simulink model "untitled55"  (R2016a)
settings: Solver=VariableStepAuto  StartTime=0.0  StopTime=1  RelTol=1e-3
settings Model: Creator=liaoyiqi  LastModifiedBy=liaoyiqi

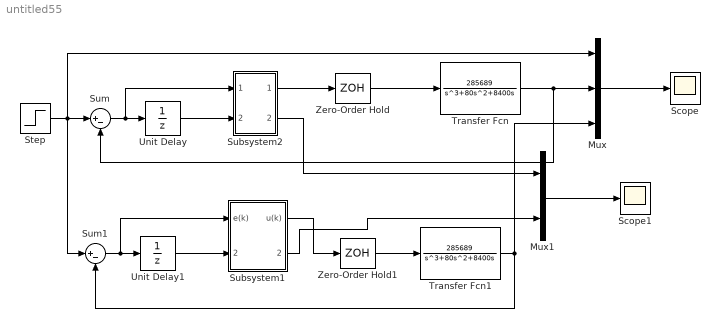
== system untitled55 ==
  Mux : Mux  Inputs=3
  Mux1 : Mux  Inputs=2
  Scope : Scope
  Scope1 : Scope
  Step : Step  Time=0  After=30  SampleTime=0
  Subsystem1 : Subsystem
  Subsystem2 : Subsystem
  Sum : Sum  Inputs=|+-
  Sum1 : Sum  Inputs=|+-
  Transfer Fcn : TransferFcn  Numerator=[285689]  Denominator=[1 80 8400 0]
  Transfer Fcn1 : TransferFcn  Numerator=[285689]  Denominator=[1 80 8400 0]
  Unit Delay : UnitDelay  SampleTime=0.001
  Unit Delay1 : UnitDelay  SampleTime=0.001
  Zero-Order Hold : ZeroOrderHold  SampleTime=0.001
  Zero-Order Hold1 : ZeroOrderHold  SampleTime=0.001
  wires:
  Step/1 -> Mux/1, Sum1/1, Sum/1
  Sum/1 -> Subsystem2/1(In1), Unit Delay/1
  Unit Delay/1 -> Subsystem2/2(In2)
  Zero-Order Hold/1 -> Transfer Fcn/1
  Mux/1 -> Scope/1
  Transfer Fcn/1 -> Sum/2, Mux/2
  Sum1/1 -> Subsystem1/1("e(k) "), Unit Delay1/1
  Subsystem2/1(Out1) -> Zero-Order Hold/1
  Unit Delay1/1 -> Subsystem1/2(e(k-1))
  Zero-Order Hold1/1 -> Transfer Fcn1/1
  Mux1/1 -> Scope1/1
  Subsystem2/2(Out2) -> Mux1/1
  Transfer Fcn1/1 -> Sum1/2, Mux/3
  Subsystem1/1(u(k)) -> Zero-Order Hold1/1
  Subsystem1/2(Out2) -> Mux1/2

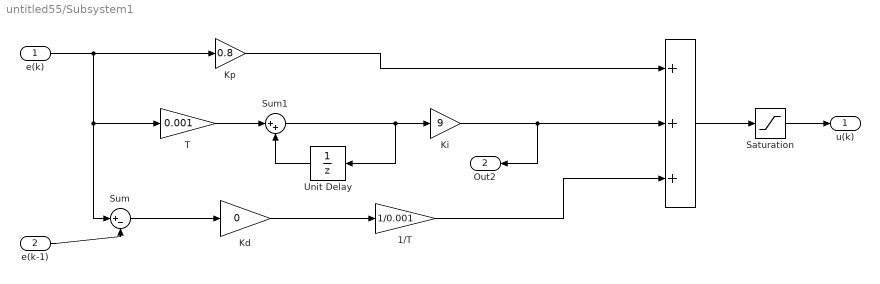
== system untitled55/Subsystem1 ==
  "e(k) " : Inport
  e(k-1) : Inport  Port=2
  " " : Sum  Inputs=+++
  1/T : Gain  Gain=1/0.001
  Kd : Gain  Gain=0
  Ki : Gain  Gain=9
  Kp : Gain  Gain=0.8
  Saturation : Saturate  UpperLimit=10  LowerLimit=-10
  Sum : Sum  Inputs=|+-
  Sum1 : Sum  Inputs=|++
  T : Gain  Gain=0.001
  Unit Delay : UnitDelay  SampleTime=0.001
  u(k) : Outport
  Out2 : Outport  Port=2
  wires:
  Sum1/1 -> Unit Delay/1, Ki/1
  Kd/1 -> 1/T/1
  Sum/1 -> Kd/1
  Unit Delay/1 -> Sum1/2
  "e(k) "/1 -> Sum/1, T/1, Kp/1
  T/1 -> Sum1/1
  1/T/1 -> " "/3
  e(k-1)/1 -> Sum/2
  Ki/1 -> Out2/1, " "/2
  Kp/1 -> " "/1
  " "/1 -> Saturation/1
  Saturation/1 -> u(k)/1

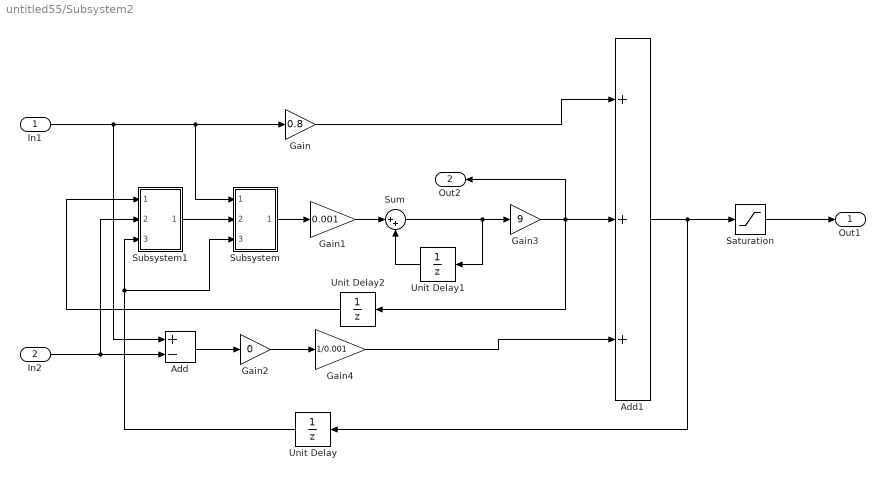
== system untitled55/Subsystem2 ==
  In1 : Inport
  In2 : Inport  Port=2
  Add : Sum  Inputs=+-
  Add1 : Sum  Inputs=+++
  Gain : Gain  Gain=0.8
  Gain1 : Gain  Gain=0.001
  Gain2 : Gain  Gain=0
  Gain3 : Gain  Gain=9
  Gain4 : Gain  Gain=1/0.001
  Saturation : Saturate  UpperLimit=10  LowerLimit=-10
  Subsystem : Subsystem
  Subsystem1 : Subsystem
  Sum : Sum  Inputs=|++
  Unit Delay : UnitDelay  SampleTime=0.001
  Unit Delay1 : UnitDelay  SampleTime=0.001
  Unit Delay2 : UnitDelay  SampleTime=0.001
  Out1 : Outport
  Out2 : Outport  Port=2
  wires:
  Sum/1 -> Unit Delay1/1, Gain3/1
  In2/1 -> Subsystem1/2(In2), Add/2
  Unit Delay/1 -> Subsystem/3(In3), Subsystem1/3(In3)
  Unit Delay1/1 -> Sum/2
  Unit Delay2/1 -> Subsystem1/1(In1)
  Add1/1 -> Unit Delay/1, Saturation/1
  In1/1 -> Subsystem/1(In1), Gain/1, Add/1
  Gain4/1 -> Add1/3
  Gain2/1 -> Gain4/1
  Add/1 -> Gain2/1
  Saturation/1 -> Out1/1
  Subsystem1/1(Out1) -> Subsystem/2(In2)
  Gain3/1 -> Out2/1, Unit Delay2/1, Add1/2
  Gain1/1 -> Sum/1
  Gain/1 -> Add1/1
  Subsystem/1(Out1) -> Gain1/1

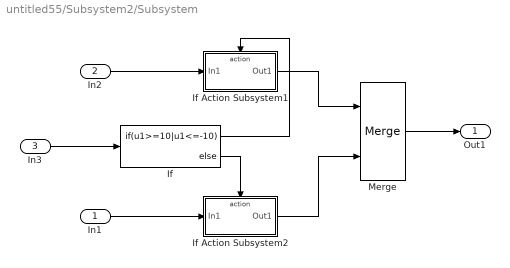
== system untitled55/Subsystem2/Subsystem ==
  In1 : Inport
  In2 : Inport  Port=2
  In3 : Inport  Port=3
  If : If  IfExpression=u1>=10|u1<=-10
  If Action Subsystem1 : Subsystem  TreatAsAtomicUnit=on
  If Action Subsystem2 : Subsystem  TreatAsAtomicUnit=on
  Merge : Merge
  Out1 : Outport
  wires:
  If/2 -> If Action Subsystem2/Action
  In1/1 -> If Action Subsystem2/1(In1)
  In2/1 -> If Action Subsystem1/1(In1)
  In3/1 -> If/1
  If Action Subsystem2/1(Out1) -> Merge/2
  Merge/1 -> Out1/1
  If Action Subsystem1/1(Out1) -> Merge/1
  If/1 -> If Action Subsystem1/Action

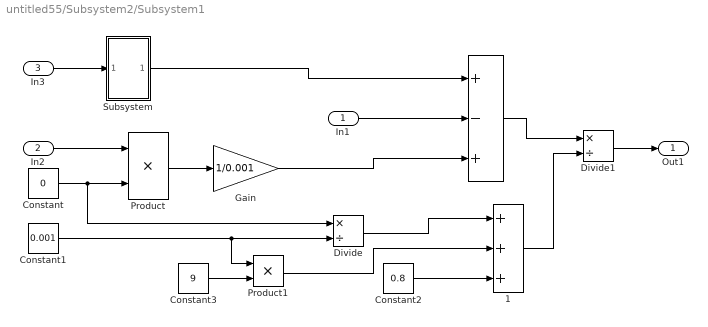
== system untitled55/Subsystem2/Subsystem1 ==
  In1 : Inport
  In2 : Inport  Port=2
  In3 : Inport  Port=3
  " " : Sum  Inputs=+-+
  " 1" : Sum  Inputs=+++
  Constant : Constant  Value=0
  Constant1 : Constant  Value=0.001
  Constant2 : Constant  Value=0.8
  Constant3 : Constant  Value=9
  Divide : Product  Inputs=*/
  Divide1 : Product  Inputs=*/
  Gain : Gain  Gain=1/0.001
  Product : Product
  Product1 : Product
  Subsystem : Subsystem
  Out1 : Outport
  wires:
  Subsystem/1(Out1) -> " "/1
  In1/1 -> " "/2
  Divide/1 -> " 1"/1
  In3/1 -> Subsystem/1(In1)
  Constant2/1 -> " 1"/3
  Constant1/1 -> Product1/1, Divide/2
  Product1/1 -> " 1"/2
  " "/1 -> Divide1/1
  Product/1 -> Gain/1
  Constant3/1 -> Product1/2
  " 1"/1 -> Divide1/2
  Gain/1 -> " "/3
  Divide1/1 -> Out1/1
  Constant/1 -> Divide/1, Product/2
  In2/1 -> Product/1

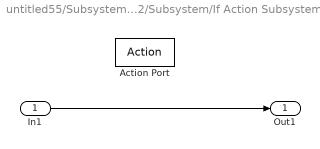
== system untitled55/Subsystem2/Subsystem/If Action Subsystem1 ==
  In1 : Inport
  Action Port : ActionPort  ActionType=then
  Out1 : Outport
  wires:
  In1/1 -> Out1/1

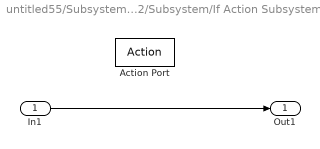
== system untitled55/Subsystem2/Subsystem/If Action Subsystem2 ==
  In1 : Inport
  Action Port : ActionPort  ActionType=else
  Out1 : Outport
  wires:
  In1/1 -> Out1/1

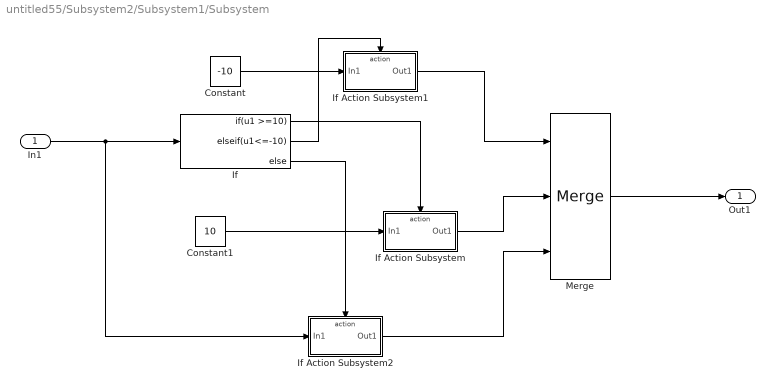
== system untitled55/Subsystem2/Subsystem1/Subsystem ==
  In1 : Inport
  Constant : Constant  Value=-10
  Constant1 : Constant  Value=10
  If : If  IfExpression=u1 >=10  ElseIfExpressions=u1<=-10
  If Action Subsystem : Subsystem  TreatAsAtomicUnit=on
  If Action Subsystem1 : Subsystem  TreatAsAtomicUnit=on
  If Action Subsystem2 : Subsystem  TreatAsAtomicUnit=on
  Merge : Merge  Inputs=3
  Out1 : Outport
  wires:
  If Action Subsystem1/1(Out1) -> Merge/1
  If Action Subsystem/1(Out1) -> Merge/2
  If/1 -> If Action Subsystem/Action
  In1/1 -> If Action Subsystem2/1(In1), If/1
  If/3 -> If Action Subsystem2/Action
  Constant1/1 -> If Action Subsystem/1(In1)
  If/2 -> If Action Subsystem1/Action
  If Action Subsystem2/1(Out1) -> Merge/3
  Constant/1 -> If Action Subsystem1/1(In1)
  Merge/1 -> Out1/1

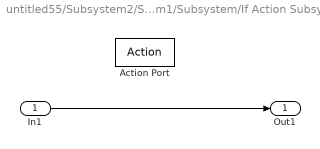
== system untitled55/Subsystem2/Subsystem1/Subsystem/If Action Subsystem ==
  In1 : Inport
  Action Port : ActionPort  ActionType=then
  Out1 : Outport
  wires:
  In1/1 -> Out1/1

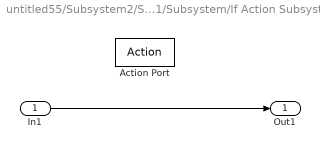
== system untitled55/Subsystem2/Subsystem1/Subsystem/If Action Subsystem1 ==
  In1 : Inport
  Action Port : ActionPort  ActionType=elseif
  Out1 : Outport
  wires:
  In1/1 -> Out1/1

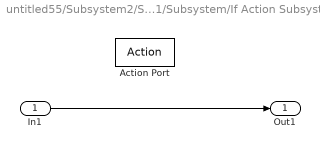
== system untitled55/Subsystem2/Subsystem1/Subsystem/If Action Subsystem2 ==
  In1 : Inport
  Action Port : ActionPort  ActionType=else
  Out1 : Outport
  wires:
  In1/1 -> Out1/1
